simulink model "smart_system"  (R2021a)
settings: Solver=VariableStepAuto  StartTime=0.0  StopTime=100.0  RelTol=1e-3
undefined symbols (not defined in the file or in its folder): control_net, sensor_model
libraries: simulink x1
settings Model: Creator=Asus  LastModifiedBy=Asus

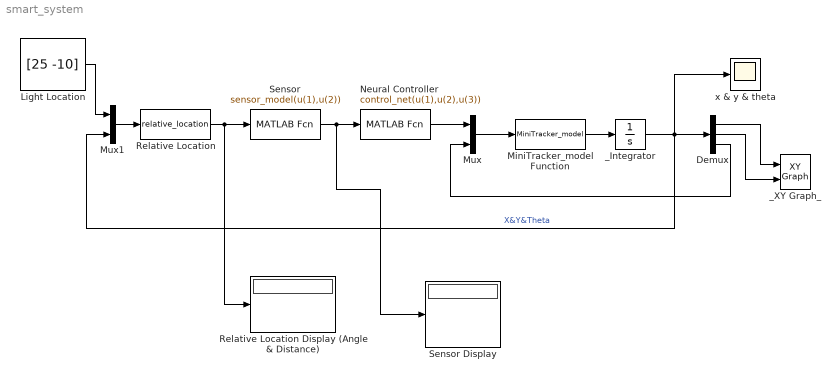
== system smart_system ==
  Demux : Demux  Outputs=3
  Light Location : Constant  Value=[25 -10]
  MiniTracker_model Function : MATLABFcn  MATLABFcn=MiniTracker_model
  Mux : Mux  Inputs=2
  Mux1 : Mux  Inputs=2
  Neural Controller : MATLABFcn  MATLABFcn=control_net(u(1),u(2),u(3))
  Relative Location : MATLABFcn  MATLABFcn=relative_location
  Relative Location Display (Angle & Distance) : Display
  Sensor : MATLABFcn  MATLABFcn=sensor_model(u(1),u(2))
  Sensor Display : Display
  _Integrator : Integrator  InitialCondition=[0 0 pi/2]
  _XY Graph_ : simulink/Sinks/XY Graph  xmin=-30  xmax=30  ymin=-30  ymax=30  st=-1
  x & y & theta : Scope
  wires:
  MiniTracker_model Function/1 -> _Integrator/1
  Mux/1 -> MiniTracker_model Function/1
  Neural Controller/1 -> Mux/1
  Demux/1 -> _XY Graph_/1
  Demux/2 -> _XY Graph_/2
  Demux/3 -> Mux/2
  Sensor/1 -> Sensor Display/1, Neural Controller/1
  Relative Location/1 -> Relative Location Display (Angle & Distance)/1, Sensor/1
  Mux1/1 -> Relative Location/1
  Light Location/1 -> Mux1/1
  _Integrator/1 -> Mux1/2, Demux/1, x & y & theta/1  "X&Y&Theta"
